simulink model "pos_cont"  (R2014a)
settings: Solver=FixedStepDiscrete  StartTime=0.0  StopTime=inf  FixedStep=sample_time  RelTol=1e-3
values from neighbouring files (symbols this model uses):
  aamp = 0.4    [pos_cont_params.m]
  aoffset = pi    (= 3.14159265359)    [pos_cont_params.m]
  daamp = 0.3    [pos_cont_params.m]
  daoffset = 0.6    [pos_cont_params.m]
  hip_d = 10    [pos_cont_params.m]
  hip_p = 1500    [pos_cont_params.m]
  hip_sat = 60    [pos_cont_params.m]
  leg_d = 40    [pos_cont_params.m]
  leg_p = 500    [pos_cont_params.m]
  leg_sat = 120    [pos_cont_params.m]
  sat_estops = false    [pos_cont_params.m]
undefined symbols (not defined in the file or in its folder): DiscIntNeverNeededParam
libraries: slrtlib x5
settings Model: SimulationMode=external  BufferReuse=off  Creator=wmartin  LastModifiedBy=drl
settings SolverCC: EnableConcurrentExecution=on
settings DataIOCC: MaxDataPoints=1000000000  SaveFormat=StructureWithTime  SaveOutput=off  SaveTime=off
settings OptimizationCC: BlockReduction=off  OptimizeBlockIOStorage=off  BufferReuse=off  GlobalBufferReuse=off  ExpressionFolding=off  ExpressionDepthLimit=2147483647  LocalBlockOutputs=off  SimCompilerOptimization=On
settings DebuggingCC: UnderspecifiedInitializationDetection=Classic  StateNameClashWarn=warning
settings HardwareCC: ProdIntDivRoundTo=Zero  ProdEndianess=LittleEndian  ProdHWDeviceType=Generic->32-bit x86 compatible
settings ModelReferenceCC: UpdateModelReferenceTargets=IfOutOfDate  ModelReferenceNumInstancesAllowed=Single  ModelReferenceMinAlgLoopOccurrences=on
settings RTWCC: SystemTargetFile=slrt.tlc  TemplateMakefile=slrt_default_tmf  Description=Simulink Real-Time  RTWVerbose=off  ProcessScript=slrt_make_rtw_hook  RTWCompilerOptimization=On
settings SimulinkRealTimeCC: GeneratePreprocessorConditionals=Disable all  EnableShiftOperators=on  RL32LogBufSizeModifier=100000000

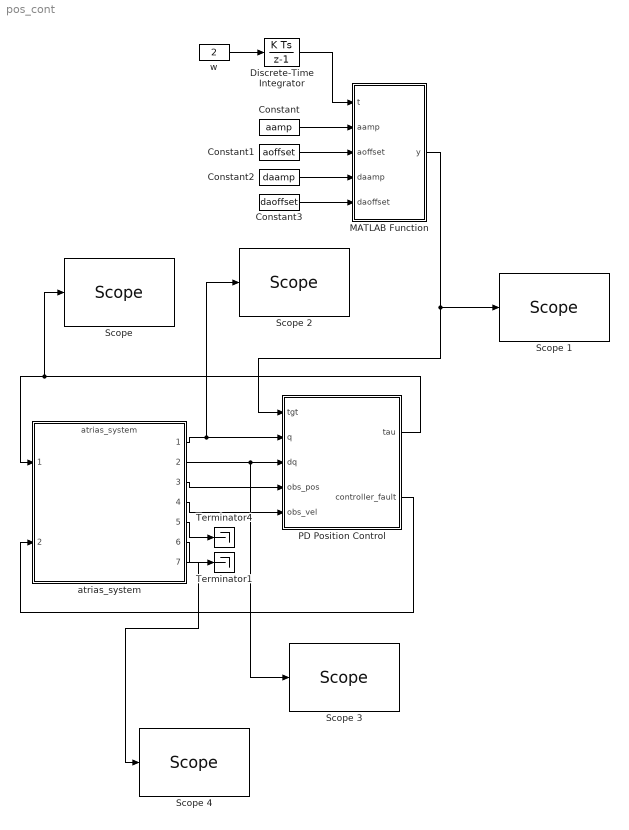
== system pos_cont ==
  Constant : Constant  Value=aamp
  Constant1 : Constant  Value=aoffset
  Constant2 : Constant  Value=daamp
  Constant3 : Constant  Value=daoffset
  Discrete-Time Integrator : DiscreteIntegrator  SampleTime=-1  ICPrevOutput=DiscIntNeverNeededParam  ICPrevScaledInput=DiscIntNeverNeededParam
  MATLAB Function : MATLAB Function  TreatAsAtomicUnit=on
  PD Position Control : MATLAB Function  TreatAsAtomicUnit=on
  "Scope " : slrtlib/Displays and Logging/Scope   scopeno=1  scopetype=Target  autostart=on  viewmode=Numerical  formatstr='%15.6f'  grid=on  ylimits=[0,0]  nosamples=100  noprepostsamples=0  interleave=1  triggermode=FreeRun  triggersignal=1  trigsignalfromport=off  triggerlevel=0.0  triggerslope=Either  triggerscope=1  triggersample=0  filename=data.dat  mode=Lazy  writesize=512  autorestart=off  dynamicfilemode=off  maxwritefilesize=512*1024^2
  Scope 1 : slrtlib/Displays and Logging/Scope   scopeno=2  scopetype=Target  autostart=on  viewmode=Graphical rolling  formatstr='%15.6f'  grid=on  ylimits=[0,0]  nosamples=2000  noprepostsamples=0  interleave=1  triggermode=FreeRun  triggersignal=1  trigsignalfromport=off  triggerlevel=0.0  triggerslope=Either  triggerscope=1  triggersample=0  filename=data.dat  mode=Lazy  writesize=512  autorestart=off  dynamicfilemode=off  maxwritefilesize=512*1024^2
  Scope 2 : slrtlib/Displays and Logging/Scope   scopeno=3  scopetype=Target  autostart=on  viewmode=Numerical  formatstr='%15.6f'  grid=on  ylimits=[0,0]  nosamples=100  noprepostsamples=0  interleave=1  triggermode=FreeRun  triggersignal=1  trigsignalfromport=off  triggerlevel=0.0  triggerslope=Either  triggerscope=1  triggersample=0  filename=data.dat  mode=Lazy  writesize=512  autorestart=off  dynamicfilemode=off  maxwritefilesize=512*1024^2
  Scope 3 : slrtlib/Displays and Logging/Scope   scopeno=4  scopetype=Target  autostart=on  viewmode=Graphical rolling  formatstr='%15.6f'  grid=on  ylimits=[0,0]  nosamples=2000  noprepostsamples=0  interleave=1  triggermode=FreeRun  triggersignal=1  trigsignalfromport=off  triggerlevel=0.0  triggerslope=Either  triggerscope=1  triggersample=0  filename=data.dat  mode=Lazy  writesize=512  autorestart=off  dynamicfilemode=off  maxwritefilesize=512*1024^2
  Scope 4 : slrtlib/Displays and Logging/Scope   scopeno=5  scopetype=Target  autostart=on  viewmode=Numerical  formatstr='%15.6f'  grid=on  ylimits=[0,0]  nosamples=100  noprepostsamples=0  interleave=1  triggermode=FreeRun  triggersignal=1  trigsignalfromport=off  triggerlevel=0.0  triggerslope=Either  triggerscope=1  triggersample=0  filename=data.dat  mode=Lazy  writesize=512  autorestart=off  dynamicfilemode=off  maxwritefilesize=512*1024^2
  Terminator1 : Terminator
  Terminator4 : Terminator
  atrias_system : ModelReference  ModelNameDialog=atrias_system  SimulationMode=Normal  ModelReferenceVersion=1.1741  CopyOfModelName=atrias_system  DefaultDataLogging=on
  w : Constant  Value=2
  wires:
  PD Position Control/1(tau) -> "Scope "/1, atrias_system/1
  atrias_system/5 -> Terminator4/1
  atrias_system/6 -> Terminator1/1
  atrias_system/3 -> PD Position Control/4(obs_pos)
  atrias_system/4 -> PD Position Control/5(obs_vel)
  atrias_system/2 -> Scope 3/1, PD Position Control/3(dq)
  atrias_system/1 -> Scope 2/1, PD Position Control/2(q)
  PD Position Control/2(controller_fault) -> atrias_system/2
  MATLAB Function/1(y) -> Scope 1/1, PD Position Control/1(tgt)
  w/1 -> Discrete-Time Integrator/1
  Discrete-Time Integrator/1 -> MATLAB Function/1(t)
  Constant3/1 -> MATLAB Function/5(daoffset)
  Constant2/1 -> MATLAB Function/4(daamp)
  Constant1/1 -> MATLAB Function/3(aoffset)
  Constant/1 -> MATLAB Function/2(aamp)
  atrias_system/7 -> Scope 4/1

== matlab function pos_cont/MATLAB Function ==
  data: t input; y output; aamp input; aoffset input; daamp input; daoffset input
function y = fcn(t, aamp, aoffset, daamp, daoffset)
%#codegen

y = [aamp * sin(t) + aoffset - (daoffset + daamp * sin(t + pi/2));
    aamp * sin(t) + aoffset + (daoffset + daamp * sin(t + pi/2));
    0;
    aamp * sin(t + pi) + aoffset - (daoffset + daamp * sin(t + 3*pi/2));
    aamp * sin(t + pi) + aoffset + (daoffset + daamp * sin(t + 3*pi/2));
    0];

== matlab function pos_cont/PD Position Control ==
  data: tgt input; tau output; q input; dq input; obs_pos input; obs_vel input; hip_sat parameter; leg_sat parameter; leg_p parameter; leg_d parameter; hip_p parameter; hip_d parameter; sat_estops parameter boolean; controller_fault output boolean
function [tau,controller_fault] = fcn(tgt, q, dq, obs_pos, obs_vel, hip_sat, leg_sat, leg_p, leg_d, hip_p, hip_d, sat_estops)
%#codegen

% Grab the motor positions and velocities in the same order as tau
% mot_q  = [ obs_pos([1 2])';  q(9)
%            obs_pos([3 4])';  q(10) ];
mot_q  = q([2, 4, 9, 6, 8, 10]);

% mot_dq = [ obs_vel([1 2])'; dq(9)
%            obs_vel([3 4])'; dq(10) ];
mot_dq = dq([2, 4, 9, 6, 8, 10]);

% Do the control
tau = [leg_p; leg_p; hip_p; leg_p; leg_p; hip_p] .* (tgt - mot_q) - ...
      [leg_d; leg_d; hip_d; leg_d; leg_d; hip_d] .* mot_dq;

% Apply the saturation limits
all_sats  = [leg_sat; leg_sat; hip_sat; leg_sat; leg_sat; hip_sat];
tau_unsat = tau;
tau       = min(tau,  all_sats);
tau       = max(tau, -all_sats);

% Check if any saturations have been hit. If so, then possibly transmit a
% controller fault
controller_fault = sat_estops & any(tau ~= tau_unsat);
